simulink model "Simulation_Pendulum"  (R2021a)
settings: Solver=VariableStepAuto  StartTime=0.0  StopTime=10  FixedStep=0.01  RelTol=1e-3
values from neighbouring files (symbols this model uses):
  b = 0.0    (= 0)    [Init_Setup_LQRArd.m]
  c = 1.91    [Init_Setup_LQRArd.m]
  g = 9.81    [Init_Setup_LQRArd.m]
  I = 0.00527    [Init_Setup_LQRArd.m]
  l = 0.26322    [Init_Setup_LQRArd.m]
  M = 0.25    [Init_Setup_LQRArd.m]
  m = 0.0693    [Init_Setup_LQRArd.m]
settings Model: Creator=jitendra  LastModifiedBy=M7540
settings SolverCC: AlgebraicLoopSolver=LineSearch
settings DataIOCC: ExternalInput=getinputstruct(op_trim1)  InitialState=getstatestruct(op_trim1)  ReturnWorkspaceOutputs=off
settings DebuggingCC: SFMachineParentedDataDiag=warning  ArithmeticOperatorsInVariantConditions=warning
settings SFSimCC: SimUseLocalCustomCode=off  CustomCodeUndefinedFunction=UseInterfaceOnly
settings RTWCC: RTWUseLocalCustomCode=off

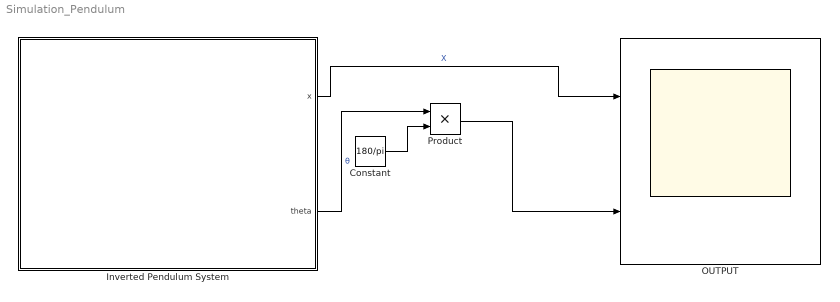
== system Simulation_Pendulum ==
  Constant : Constant  Value=180/pi
  Inverted Pendulum System : Subsystem
      mask Display: image('C:\Users\M7540\Desktop\ip\Image\mô hình toán học con lắc.jpg'); % Use "Edit Image" on toolstrip to change.
  OUTPUT : Scope  NumInputPorts=2
  Product : Product
  wires:
  Inverted Pendulum System/1(x) -> OUTPUT/1  "X"
  Inverted Pendulum System/2(theta) -> Product/1  "θ"
  Constant/1 -> Product/2
  Product/1 -> OUTPUT/2

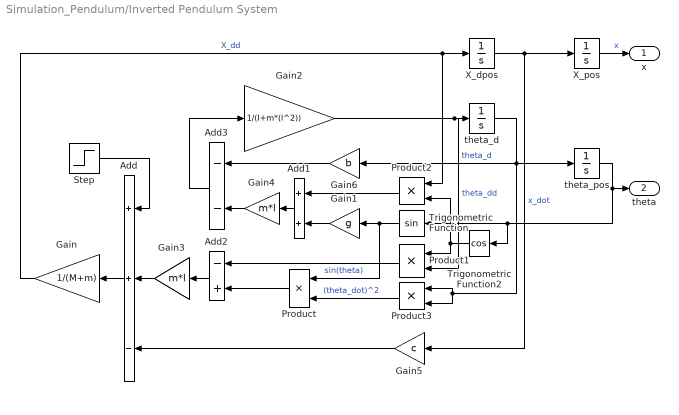
== system Simulation_Pendulum/Inverted Pendulum System ==
  Add : Sum  Inputs=++-
  Add1 : Sum
  Add2 : Sum  Inputs=-+
  Add3 : Sum  Inputs=--
  Gain : Gain  Gain=1/(M+m)
  Gain1 : Gain  Gain=g
  Gain2 : Gain  Gain=1/(I+m*(l^2))
  Gain3 : Gain  Gain=m*l
  Gain4 : Gain  Gain=m*l
  Gain5 : Gain  Gain=c
  Gain6 : Gain  Gain=b
  Product{,1..3} (4 alike) : Product
  Step : Step  Before=1  After=0  OutDataTypeStr=single  SampleTime=0
  Trigonometric Function : Trigonometry
  Trigonometric Function2 : Trigonometry  Operator=cos
  X_dpos : Integrator  InitialCondition=0.01
  X_pos : Integrator  InitialCondition=0.0
  theta_d : Integrator
  theta_pos : Integrator  InitialCondition=-0.001*(pi/180)
  x : Outport  VectorParamsAs1DForOutWhenUnconnected=off
  theta : Outport  Port=2  VectorParamsAs1DForOutWhenUnconnected=off
  wires:
  Gain5/1 -> Add/3
  Add2/1 -> Gain3/1
  Add3/1 -> Gain2/1
  Trigonometric Function2/1 -> Product2/2, Product1/1
  Trigonometric Function/1 -> Product/1, Gain1/1  "sin(theta)"
  Gain3/1 -> Add/2
  theta_d/1 -> Product3/2, Product3/1, Gain6/1, theta_pos/1  "theta_d"
  Product2/1 -> Add1/1
  Product/1 -> Add2/2
  Gain4/1 -> Add3/2
  Product3/1 -> Product/2  "(theta_dot)^2"
  X_pos/1 -> x/1  "x"
  Product1/1 -> Add2/1
  Gain/1 -> X_dpos/1, Product2/1  "X_dd"
  Add/1 -> Gain/1
  Gain2/1 -> Product1/2, theta_d/1  "theta_dd"
  Gain6/1 -> Add3/1
  theta_pos/1 -> Trigonometric Function2/1, Trigonometric Function/1, theta/1
  Gain1/1 -> Add1/2
  X_dpos/1 -> X_pos/1, Gain5/1  "x_dot"
  Add1/1 -> Gain4/1
  Step/1 -> Add/1
